simulink model "untitled"  (R2019a)
settings: Solver=VariableStepAuto  StartTime=0.0  StopTime=10.0  RelTol=1e-3
values from neighbouring files (symbols this model uses):
  KK7 = lqr(A,B,Q,R)    [thongsoxe2banh.m]
settings Model: Creator=Duong  LastModifiedBy=Duong

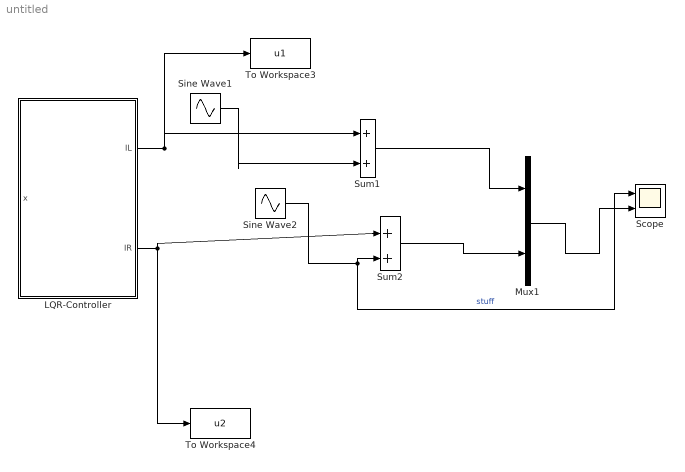
== system untitled ==
  LQR-Controller : Subsystem
  Mux1 : Mux  Inputs=2
  Scope : Scope  NumInputPorts=2
  Sine Wave1 : Sin  Amplitude=0  Bias=.2  Phase=pi/6  SampleTime=0
  Sine Wave2 : Sin  Amplitude=0  Bias=-.2  Frequency=2  Phase=pi/4  SampleTime=0
  Sum1 : Sum  Inputs=|++
  Sum2 : Sum  Inputs=|++
  To Workspace3 : ToWorkspace  VariableName=u1  SaveFormat=Timeseries  SampleTime=-1
  To Workspace4 : ToWorkspace  VariableName=u2  SaveFormat=Timeseries  SampleTime=-1
  wires:
  Sum2/1 -> Mux1/2
  Sine Wave2/1 -> Scope/1, Sum2/2  "stuff"
  Sine Wave1/1 -> Sum1/2
  Sum1/1 -> Mux1/1
  LQR-Controller/2(IR) -> To Workspace4/1, Sum2/1
  LQR-Controller/1(IL) -> Sum1/1, To Workspace3/1
  Mux1/1 -> Scope/2
  ? -> LQR-Controller/1(x)

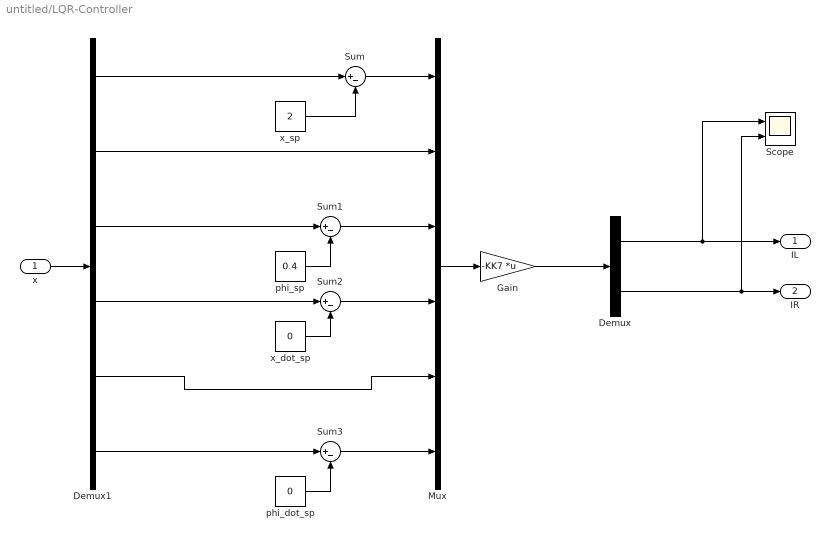
== system untitled/LQR-Controller ==
  x : Inport
  Demux : Demux  Outputs=2
  Demux1 : Demux  Outputs=6
  Gain : Gain  Gain=-KK7  Multiplication=Matrix(K*u)
  Mux : Mux  Inputs=6
  Scope : Scope  NumInputPorts=2
  Sum{,1..3} (4 alike) : Sum  Inputs=|+-
  "phi_dot_sp " : Constant  Value=0
  "phi_sp " : Constant  Value=0.4
  "x_dot_sp " : Constant  Value=0
  "x_sp " : Constant  Value=2
  IL : Outport
  IR : Outport  Port=2
  wires:
  Sum/1 -> Mux/1
  Demux1/1 -> Sum/1
  Demux1/2 -> Mux/2
  Sum1/1 -> Mux/3
  Demux1/3 -> Sum1/1
  "phi_sp "/1 -> Sum1/2
  Sum2/1 -> Mux/4
  Demux1/4 -> Sum2/1
  "x_dot_sp "/1 -> Sum2/2
  Demux1/6 -> Sum3/1
  "phi_dot_sp "/1 -> Sum3/2
  Sum3/1 -> Mux/6
  Demux1/5 -> Mux/5
  Mux/1 -> Gain/1
  Gain/1 -> Demux/1
  Demux/2 -> Scope/2, IR/1
  Demux/1 -> Scope/1, IL/1
  "x_sp "/1 -> Sum/2
  x/1 -> Demux1/1
